simulink model "segway_control"  (R2025b)
settings: Solver=ode45  StartTime=0.0  StopTime=5  RelTol=1e-6  AbsTol=1e-8
values from neighbouring files (symbols this model uses):
  K = place(A, B, polos_deseados)    [segway_controlador.m]
  params_vec = [p.M; p.m; p.r; p.d; p.l; p.g;                p.Icy; p.Icz; p.Icx; p.Iw; p.Iwz; p.alpha_m; p.beta_m]    [segway_sim_lazo_abierto.m]
settings Model: Creator=crist  LastModifiedBy=crist
settings DataIOCC: SaveFormat=Array

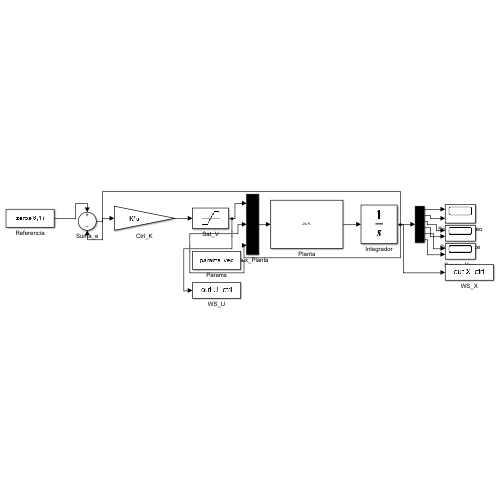
[thumbnail: Simulink's stored preview of the top-level diagram]
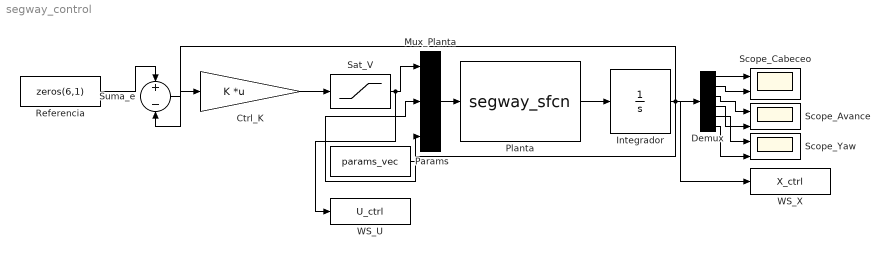
== system segway_control ==
  Ctrl_K : Gain  Gain=K  Multiplication=Matrix(K*u)
  Demux : Demux  Outputs=6
  Integrador : Integrator  InitialCondition=[0.05; 0; 0; 0; 0; 0]
  Mux_Planta : Mux  Inputs=3
  Params : Constant  Value=params_vec
  Planta : MATLABFcn  MATLABFcn=segway_sfcn  OutputDimensions=6
  Referencia : Constant  Value=zeros(6,1)
  Sat_V : Saturate  UpperLimit=12  LowerLimit=-12
  Scope_Avance : Scope  NumInputPorts=2
  Scope_Cabeceo : Scope  NumInputPorts=2
  Scope_Yaw : Scope  NumInputPorts=2
  Suma_e : Sum  Inputs=+-
  WS_U : ToWorkspace  VariableName=U_ctrl  SampleTime=-1
  WS_X : ToWorkspace  VariableName=X_ctrl  SampleTime=-1
  wires:
  Referencia/1 -> Suma_e/1
  Suma_e/1 -> Ctrl_K/1
  Ctrl_K/1 -> Sat_V/1
  Sat_V/1 -> Mux_Planta/1, WS_U/1
  Params/1 -> Mux_Planta/2
  Integrador/1 -> Mux_Planta/3, Suma_e/2, Demux/1, WS_X/1
  Mux_Planta/1 -> Planta/1
  Planta/1 -> Integrador/1
  Demux/1 -> Scope_Cabeceo/1
  Demux/2 -> Scope_Cabeceo/2
  Demux/3 -> Scope_Avance/1
  Demux/4 -> Scope_Avance/2
  Demux/5 -> Scope_Yaw/1
  Demux/6 -> Scope_Yaw/2
